simulink model "hr_sliding_mode_control"  (R2024b)
settings: Solver=VariableStepAuto  StartTime=0.0  StopTime=T  FixedStep=1e-3  MaxStep=1e-3  RelTol=1e-5  AbsTol=1e-7
values from neighbouring files (symbols this model uses):
  a = 1    [bifurcation_diagram.m]    (also in equilibria.m; flow.m; flow_analysis.m; linear_analysis.m)
  b = 3    [bifurcation_diagram.m]    (also in equilibria.m; flow.m; flow_analysis.m; linear_analysis.m = linspace(0, 10, 100))
  c = 1    [bifurcation_diagram.m]    (also in equilibria.m; flow.m; flow_analysis.m; linear_analysis.m)
  d = 5    [bifurcation_diagram.m]    (also in equilibria.m; flow.m; flow_analysis.m; linear_analysis.m)
  I = linspace(1.2, 3.5, 1000)    [bifurcation_diagram.m]    (also in equilibria.m = 1.309; flow.m = 1.3059; linear_analysis.m = 2; params.m = 1.28)
  k_smc = 1.2    [params.m]
  p1 = plot(real(current_lambdas(:, k)), imag(current_lambdas(:, k)), 'b.', 'MarkerSize', 4)    [linear_analysis.m]    (also in params.m = 1.33)
  r = 0.003    [bifurcation_diagram.m]    (also in equilibria.m; flow.m; flow_analysis.m; linear_analysis.m = 0.001)
  regulation = 0    [params.m]    (also in plot_sim_reg.m = 1; plot_sim_reg_disturbance.m = 1; plot_sim_reg_uncertainties.m = 1; plot_sim_track.m)
  s = 4    [bifurcation_diagram.m]    (also in equilibria.m; flow.m; flow_analysis.m; linear_analysis.m)
  uncertainty = 0    [params.m]    (also in plot_sim_reg.m; plot_sim_reg_disturbance.m; plot_sim_reg_uncertainties.m = 1; plot_sim_track.m)
  x_0 = [0.1; 0.1; 0.1]    [bifurcation_diagram.m]    (also in flow.m = x_0_generic; params.m; plot_sim_track.m = hr_equilibria(a,b,c,d,s,x_r,I); plot_sim_track_disturbance.m = hr_equilibria(a,b,c,d,s,x_r,I))
  x_eq = current_eq(1, j)    [linear_analysis.m]    (also in params.m = eq(1,1); plot_sim_track.m = eq(1,1); plot_sim_track_disturbance.m = eq(1,1); plot_sim_track_uncertainties.m = eq(1,1))
  x_r = -8/5    (= -1.6)    [bifurcation_diagram.m]    (also in equilibria.m; flow.m; flow_analysis.m; linear_analysis.m)
settings Model: Creator=vincip  LastModifiedBy=vincip
settings SolverCC: InitialStep=1e-5

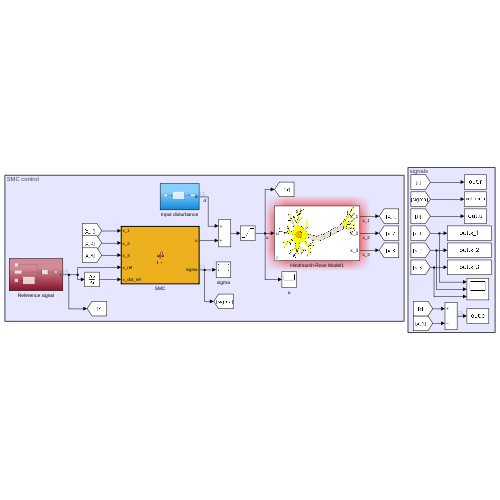
[thumbnail: Simulink's stored preview of the top-level diagram]
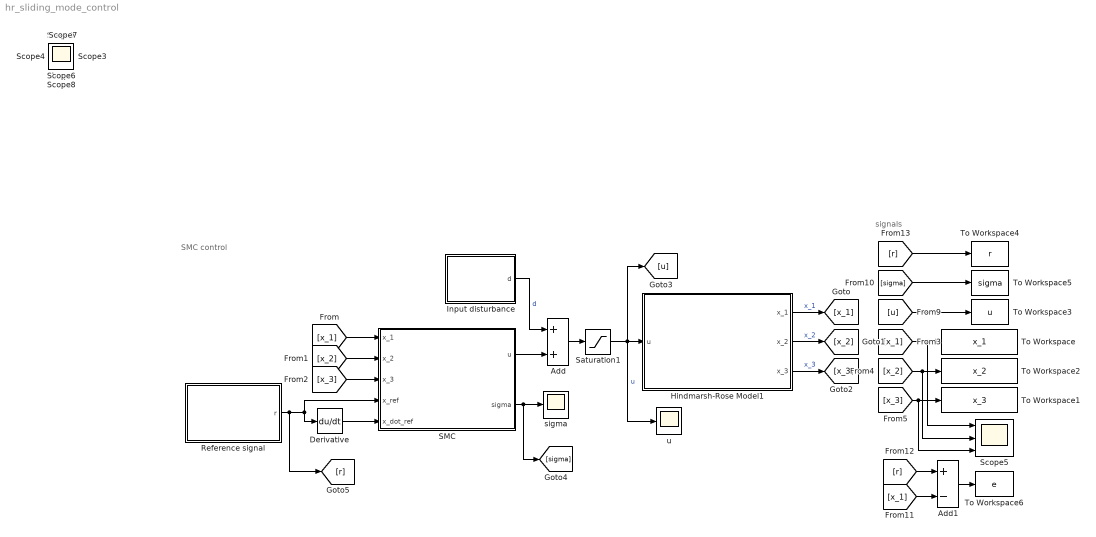
== system hr_sliding_mode_control ==
  note: signals
  note: SMC control
  Add : Sum
  Add1 : Sum  Inputs=+-
  Derivative : Derivative
  Hindmarsh-Rose Model1 : Subsystem  mask{a=a, b=b, c=c, d=d, r=r, s=s, x_r=x_r, I=I, x_0=x_0, uncertainty=uncertainty}
      mask DialogControl DescTextVar Prompt: Hindmarsh-Rose Neuronal Model with an external input u
      mask Display:
      | image('figures/neuron.jpg');
      | port_label('input', 1, 'u');
      | port_label('output', 1, 'x_1');
      | port_label('output', 2, 'x_2');
      | port_label('output', 3, 'x_3');
  Input disturbance : Subsystem
  Reference signal : Subsystem
  SMC : MATLAB Function  TreatAsAtomicUnit=on
  Saturation1 : Saturate  UpperLimit=10  LowerLimit=-10  LinearizeAsGain=off  ZeroCross=off
  Scope5 : Scope  NumInputPorts=3
  To Workspace : ToWorkspace  VariableName=x_1  SaveFormat=Timeseries  SampleTime=-1
  To Workspace1 : ToWorkspace  VariableName=x_3  SaveFormat=Timeseries  SampleTime=-1
  To Workspace2 : ToWorkspace  VariableName=x_2  SaveFormat=Timeseries  SampleTime=-1
  To Workspace3 : ToWorkspace  VariableName=u  SaveFormat=Timeseries  SampleTime=-1
  To Workspace4 : ToWorkspace  VariableName=r  SaveFormat=Timeseries  SampleTime=-1
  To Workspace5 : ToWorkspace  VariableName=sigma  SaveFormat=Timeseries  SampleTime=-1
  To Workspace6 : ToWorkspace  VariableName=e  SaveFormat=Timeseries  SampleTime=-1
  sigma : Scope
  u : Scope
  Scope{,1..4,6..8} (8 alike) : Scope
  wires:
  Hindmarsh-Rose Model1/1(x_1) -> [x_1]  "x_1"
  SMC/2(sigma) -> [sigma], sigma/1
  Derivative/1 -> SMC/5(x_dot_ref)
  Reference signal/1(r) -> [r], SMC/4(x_ref), Derivative/1
  [x_1] -> SMC/1(x_1)
  Hindmarsh-Rose Model1/2(x_2) -> [x_2]  "x_2"
  [x_2] -> SMC/2(x_2)
  Hindmarsh-Rose Model1/3(x_3) -> [x_3]  "x_3"
  [x_3] -> SMC/3(x_3)
  [x_1] -> Scope5/1, To Workspace/1
  [x_2] -> Scope5/2, To Workspace2/1
  [x_3] -> To Workspace1/1, Scope5/3
  SMC/1(u) -> Add/2
  Input disturbance/1(d) -> Add/1  "d"
  Add/1 -> Saturation1/1
  Saturation1/1 -> Hindmarsh-Rose Model1/1(u), [u], u/1  "u"
  [u] -> To Workspace3/1
  [sigma] -> To Workspace5/1
  [x_1] -> Add1/2
  [r] -> Add1/1
  [r] -> To Workspace4/1
  Add1/1 -> To Workspace6/1

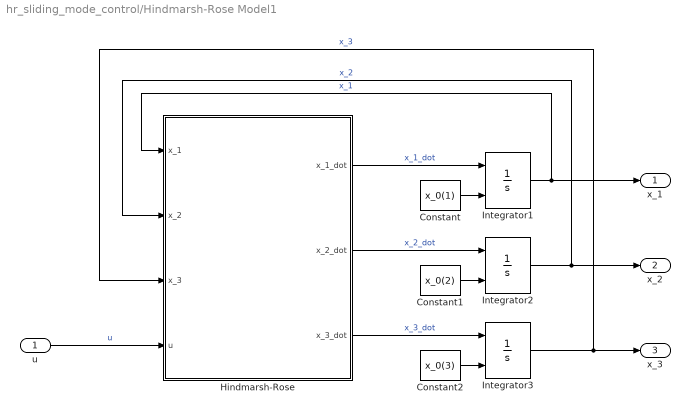
== system hr_sliding_mode_control/Hindmarsh-Rose Model1 ==
  u : Inport
  Constant : Constant  Value=x_0(1)
  Constant1 : Constant  Value=x_0(2)
  Constant2 : Constant  Value=x_0(3)
  Hindmarsh-Rose : MATLAB Function  TreatAsAtomicUnit=on
  Integrator1 : Integrator  InitialConditionSource=external  InitialCondition=x_0
  Integrator2 : Integrator  InitialConditionSource=external  InitialCondition=x_0
  Integrator3 : Integrator  InitialConditionSource=external  InitialCondition=x_0
  x_1 : Outport
  x_2 : Outport  Port=2
  x_3 : Outport  Port=3
  wires:
  Hindmarsh-Rose/2(x_2_dot) -> Integrator2/1  "x_2_dot"
  Integrator1/1 -> Hindmarsh-Rose/1(x_1), x_1/1  "x_1"
  Hindmarsh-Rose/3(x_3_dot) -> Integrator3/1  "x_3_dot"
  Integrator3/1 -> x_3/1, Hindmarsh-Rose/3(x_3)  "x_3"
  u/1 -> Hindmarsh-Rose/4(u)  "u"
  Hindmarsh-Rose/1(x_1_dot) -> Integrator1/1  "x_1_dot"
  Integrator2/1 -> Hindmarsh-Rose/2(x_2), x_2/1  "x_2"
  Constant/1 -> Integrator1/2
  Constant1/1 -> Integrator2/2
  Constant2/1 -> Integrator3/2

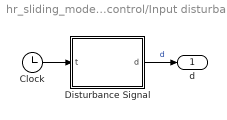
== system hr_sliding_mode_control/Input disturbance ==
  Clock : Clock
  Disturbance Signal : MATLAB Function  TreatAsAtomicUnit=on
  d : Outport
  wires:
  Clock/1 -> Disturbance Signal/1(t)
  Disturbance Signal/1(d) -> d/1  "d"

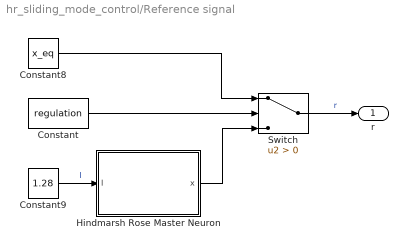
== system hr_sliding_mode_control/Reference signal ==
  Constant : Constant  Value=regulation
  Constant8 : Constant  Value=x_eq
  Constant9 : Constant  Value=1.28
  Hindmarsh Rose Master Neuron : Subsystem  mask{a=a, b=b, c=c, d=d, r=r, s=s, x_r=x_r, x_0=x_0}
      mask DialogControl DescTextVar Prompt: Hindmarsh-Rose Master neuronal model
      mask Display:
      | disp('Hindmarsh-Rose\nMaster Neuron');
      | port_label('output', 1, 'x');
      | port_label('input', 1, 'I');
  Switch : Switch  Criteria=u2 > Threshold  SaturateOnIntegerOverflow=off  InputSameDT=off
  r : Outport
  wires:
  Switch/1 -> r/1  "r"
  Constant8/1 -> Switch/1
  Constant/1 -> Switch/2
  Constant9/1 -> Hindmarsh Rose Master Neuron/1(I)  "I"
  Hindmarsh Rose Master Neuron/1(x) -> Switch/3

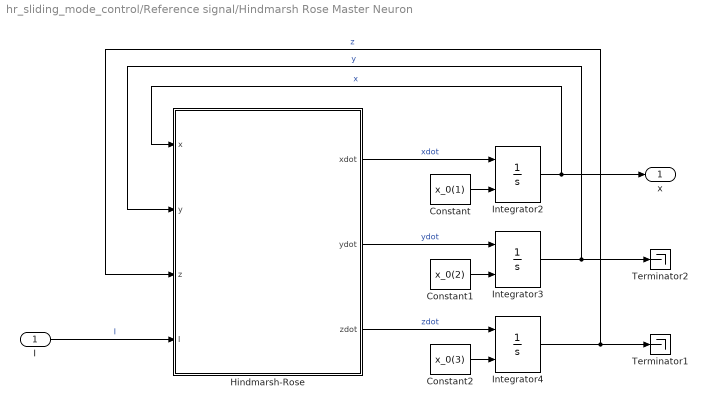
== system hr_sliding_mode_control/Reference signal/Hindmarsh Rose Master Neuron ==
  I : Inport
  Constant : Constant  Value=x_0(1)
  Constant1 : Constant  Value=x_0(2)
  Constant2 : Constant  Value=x_0(3)
  Hindmarsh-Rose : MATLAB Function  TreatAsAtomicUnit=on
  Integrator2 : Integrator  InitialConditionSource=external  InitialCondition=x_0
  Integrator3 : Integrator  InitialConditionSource=external  InitialCondition=x_0
  Integrator4 : Integrator  InitialConditionSource=external  InitialCondition=x_0
  Terminator1 : Terminator
  Terminator2 : Terminator
  x : Outport
  wires:
  Hindmarsh-Rose/1(xdot) -> Integrator2/1  "xdot"
  I/1 -> Hindmarsh-Rose/4(I)  "I"
  Integrator3/1 -> Terminator2/1, Hindmarsh-Rose/2(y)  "y"
  Hindmarsh-Rose/3(zdot) -> Integrator4/1  "zdot"
  Integrator2/1 -> x/1, Hindmarsh-Rose/1(x)  "x"
  Integrator4/1 -> Terminator1/1, Hindmarsh-Rose/3(z)  "z"
  Constant2/1 -> Integrator4/2
  Hindmarsh-Rose/2(ydot) -> Integrator3/1  "ydot"
  Constant/1 -> Integrator2/2
  Constant1/1 -> Integrator3/2

== matlab function hr_sliding_mode_control/SMC ==
  data: x_1 input; x_2 input; x_3 input; u output; x_ref input; x_dot_ref input; sigma output; a parameter; b parameter; k_smc parameter; regulation parameter; p1 parameter; I parameter
function [u, sigma] = fcn(x_1, x_2, x_3, x_ref, x_dot_ref, a, b, k_smc, regulation, p1, I)
% Define sliding function sigma based on regulation or tracking
x_1_dot = x_2 - a*x_1^3 + b*x_1^2 - x_3 + I;
if regulation == 1
    sigma = p1*(x_1 - x_ref);
    % Define control action
    u_eq = -x_2 + a*x_1^3 - b*x_1^2 + x_3 - I;
else
    sigma = p1*(x_1 - x_ref); % + p2*(x_dot - x_dot_ref) + p1*e_int;
    % Define control action
    u_eq =  x_dot_ref - x_1_dot; %- (p1/p2)*(x - x_ref) - (p1/p2)*e_int;
end

phi = 0.001;
if abs(sigma) <= phi
    u_sw = -k_smc * (sigma / phi);
else
    u_sw = -k_smc * sign(sigma);
end
% u_sw = -k_smc * sign(sigma);
% epsilon = 0.05;
% u_sw = -k_smc * tanh(sigma/epsilon);
% Control output
u = u_eq + u_sw;

== matlab function hr_sliding_mode_control/Input disturbance/Disturbance Signal ==
  data: d output; t input; choice parameter
function d = disturbance(t, choice)
% Select input disturbance based on the choice parameter
ampl = 0.5;
w = 2*pi * 0.2;
if choice == 1
    d = ampl * sin(w * t);
elseif choice == 2
    if t >= 1.0
        d = 1.0;
    else 
        d = 0.0;
    end
else
    d = 0;
end

== matlab function hr_sliding_mode_control/Hindmarsh-Rose Model1/Hindmarsh-Rose ==
  data: x_1 input; x_2 input; x_3 input; u input; x_1_dot output; x_2_dot output; x_3_dot output; a parameter; b parameter; c parameter; d parameter; s parameter; r parameter; x_r parameter; I parameter; uncertainty parameter
function [x_1_dot, x_2_dot, x_3_dot]  = hrindmarsh_rose_model(x_1, x_2, x_3, ...
    u, a, b, c, d, s, r, x_r, I, uncertainty)
    % potential uncertainty
    delta = 0.1;
    if uncertainty == 1
        a_real = a*(1 + delta);
        b_real = b*(1 + delta);
        c_real = c*(1 + delta);
        d_real = d*(1 + delta);
    else
        a_real = a;
        b_real = b;
        c_real = c;
        d_real = d;
    end
    % Neuronal model - Hindmarsh Rose
    x_1_dot = x_2 - a_real*x_1^3 + b_real*x_1^2 - x_3 + I + u;
    x_2_dot = c_real - d_real*x_1^2 - x_2;
    x_3_dot = r*(s*(x_1 - x_r) - x_3);

== matlab function hr_sliding_mode_control/Reference signal/Hindmarsh Rose Master Neuron/Hindmarsh-Rose ==
  data: x input; y input; z input; xdot output; ydot output; zdot output; a parameter; b parameter; c parameter; d parameter; s parameter; r parameter; x_r parameter; I input
function [xdot, ydot, zdot]  = hrindmarsh_rose_model(x, y, z, a, b, c, d, s, r, x_r, I)
    % Neuronal model - Hindmarsh Rose
    xdot = y - a*x^3 + b*x^2 - z + I;
    ydot = c - d*x^2 - y;
    zdot = r*(s*(x - x_r) - z);
